simulink model "h2omnix_heading"  (R2022b)
settings: Solver=ode4  StartTime=0.0  StopTime=inf  FixedStep=0.05  RelTol=1e-3
values from neighbouring files (symbols this model uses):
  nu_max = [0.5,0.5,1]'    [parameters.m]
  nu_min = -nu_max    [parameters.m]
  pcKd = pcKd.*disable    [parameters.m]
  pcKp = pcKp.*disable    [parameters.m]
  vcKi = vcKi.*disable    [parameters.m]
  vcKp = vcKp.*disable    [parameters.m]
  vcKt = vcKt.*disable    [parameters.m]
  wn = 3*wpn/2    [parameters.m]
  wpn = [1.2, 1.2, 1]'    [parameters.m]
libraries: ros2lib x4, MarineRoboticsLib x3, MarineRoboticsLibEx x1, robotcorelib x1, matrix_library x1, simulink x1
settings Model: DataDictionary=ros2lib.sldd  Creator=dnad  LastModifiedBy=dnad

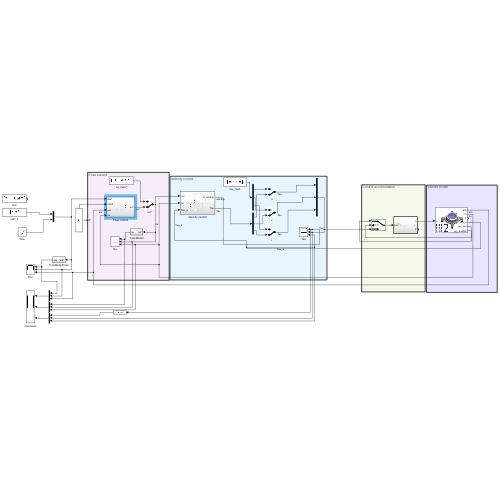
[thumbnail: Simulink's stored preview of the top-level diagram]
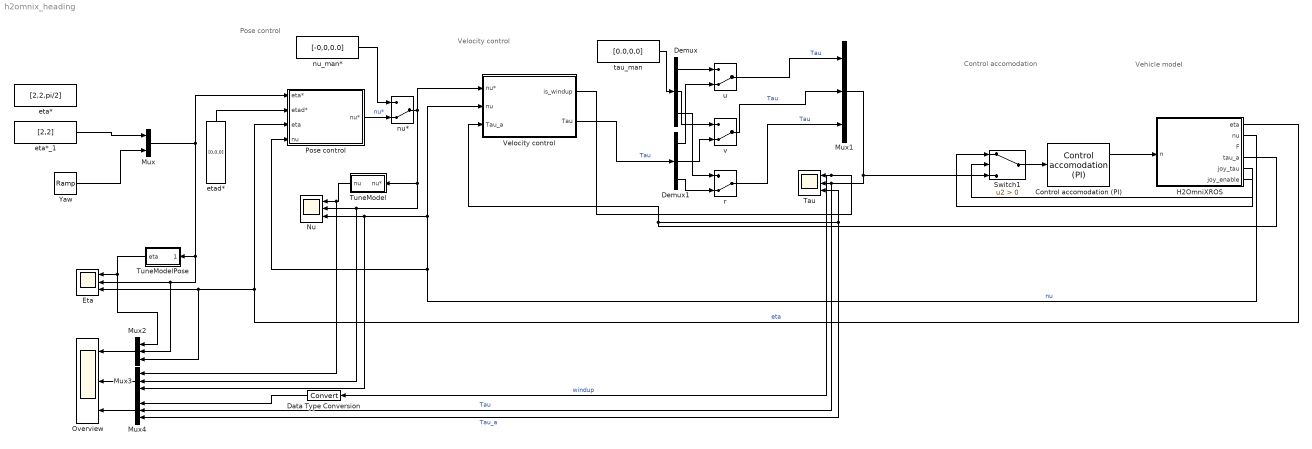
== system h2omnix_heading ==
  note: Control accomodation
  note: Vehicle model
  note: Pose control
  note: Velocity control
  Control accomodation (PI) : MarineRoboticsLibEx/Control accomodation (PI)  SystemSampleTime=-1  VariantActivationTime=update diagram  Latency=0  AutoFrameSizeCalculation=off
  Data Type Conversion : DataTypeConversion  SaturateOnIntegerOverflow=off  RndMeth=Floor
  Demux : Demux  Outputs=3
  Demux1 : Demux  Outputs=3
  Eta : Scope  NumInputPorts=3
  H2OmniXROS : Subsystem  AncestorBlock=MarineRoboticsLib/H2OmniXROS  mask{vehicle_name=krk, max_pwm=0.4, pwm_topic=/krk/pwm_out, joy_topic=/krk/joy, odometry_topic=/krk/odometry/filtered}
      mask prompts: vehicle_name "Vehicle name"; max_pwm "Maximum allowed PWM"; pwm_topic "Command"; joy_topic "Joystick"; odometry_topic "Odometry"
      mask init:
      | set_param(gcb, 'pwm_topic',strcat('/', vehicle_name, '/pwm_out'));
      |     set_param(gcb, 'odometry_topic', strcat('/', vehicle_name, '/odometry/filtered'));
      |     set_param(gcb, 'joy_topic', strcat('/', vehicle_name, '/joy'));
      settings: LibrarySourceBlock=MarineRoboticsLib/H2OmniXROS
      mask TypeOptions pwm_topic: PublishToROS/topic
      mask TypeOptions joy_topic: Subscribe2/topic
      mask TypeOptions odometry_topic: Subscribe1/topic
      mask DialogControl G1 Prompt: Topics
      mask Display: image('$imagefile'); % Use "Edit Image" on toolstrip to change.
  Mux : Mux  Inputs=2
  Mux{1..4} (4 alike) : Mux  Inputs=3
  Nu : Scope  NumInputPorts=3
  Overview : Scope  NumInputPorts=3
  Pose control : Subsystem
  Switch1 : Switch  Criteria=u2 > Threshold  SaturateOnIntegerOverflow=off  InputSameDT=off
  Tau : Scope  NumInputPorts=3
  TuneModel : Subsystem
  TuneModelPose : Subsystem
  Velocity control : Subsystem
  Yaw : simulink/Sources/Ramp  slope=0.5  start=0  InitialOutput=0
  eta* : Constant  Value=[2,2,pi/2]
  eta*_1 : Constant  Value=[2,2]
  etad* : Constant  Value=[0,0,0]
  nu* : ManualSwitch  CurrentSetting=0
  nu_man* : Constant  Value=[-0,0,0.0]
  r : ManualSwitch  CurrentSetting=0
  tau_man : Constant  Value=[0.0,0,0]
  u : ManualSwitch  CurrentSetting=0
  v : ManualSwitch  CurrentSetting=0
  wires:
  Switch1/1 -> Control accomodation (PI)/1
  Control accomodation (PI)/1 -> H2OmniXROS/1(n)
  H2OmniXROS/5(joy_tau) -> Switch1/1
  H2OmniXROS/6(joy_enable) -> Switch1/2
  TuneModelPose/1(eta) -> Mux2/1, Eta/1
  Velocity control/1(is_windup) -> Data Type Conversion/1, Tau/1  "windup"
  etad*/1 -> Pose control/2(etad*)
  Pose control/1(nu*) -> nu*/2  "nu*"
  eta*_1/1 -> Mux/1
  Mux1/1 -> Mux4/2, Tau/2, Switch1/3  "Tau"
  TuneModel/1(nu) -> Mux3/1, Nu/1
  nu_man*/1 -> nu*/1
  H2OmniXROS/1(eta) -> Pose control/3(eta), Mux2/3, Eta/3  "eta"
  H2OmniXROS/2(nu) -> Velocity control/2(nu), Mux3/3, Nu/3, Pose control/4(nu)  "nu"
  H2OmniXROS/4(tau_a) -> Velocity control/3(Tau_a), Mux4/3, Tau/3  "Tau_a"
  Yaw/1 -> Mux/2
  nu*/1 -> Mux3/2, Nu/2, TuneModel/1(nu*), Velocity control/1(nu*)
  Mux/1 -> Pose control/1(eta*), Mux2/2, Eta/2, TuneModelPose/1(eta*)
  tau_man/1 -> Demux/1
  Velocity control/2(Tau) -> Demux1/1  "Tau"
  Demux/1 -> u/1
  Demux1/1 -> u/2
  Demux/2 -> v/1
  Demux1/2 -> v/2
  Demux/3 -> r/1
  Demux1/3 -> r/2
  r/1 -> Mux1/3  "Tau"
  v/1 -> Mux1/2  "Tau"
  u/1 -> Mux1/1  "Tau"
  Mux2/1 -> Overview/1
  Mux3/1 -> Overview/2
  Mux4/1 -> Overview/3
  Data Type Conversion/1 -> Mux4/1

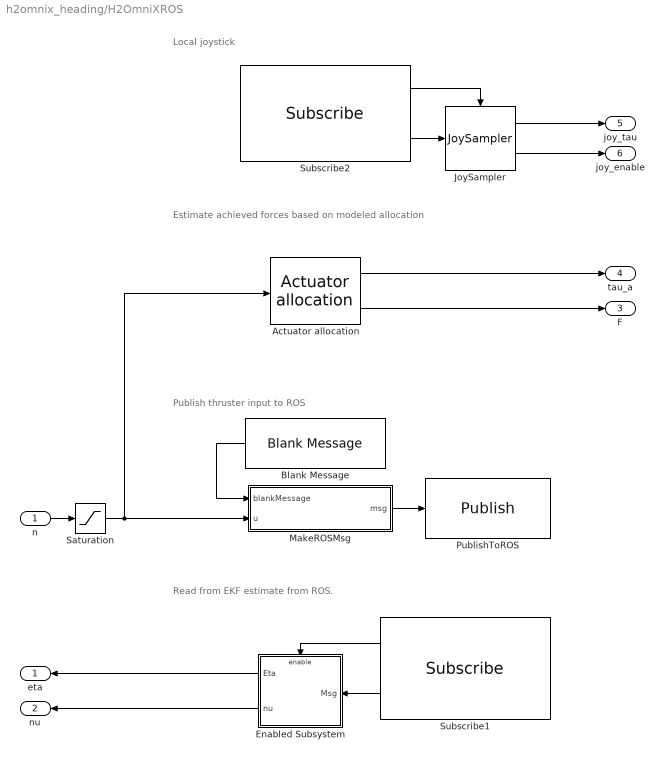
== system h2omnix_heading/H2OmniXROS ==
  note: Local joystick
  note: Read from EKF estimate from ROS.
  note: Publish thruster input to ROS
  note: Estimate achieved forces based on modeled allocation
  n : Inport
  Actuator allocation : MarineRoboticsLib/Actuator allocation  Tm=0  B="[0.25, 0.25, -0.25, -0.25; -0.25,  0.25, -0.25,  0.25; -0.25, 0.25, 0.25, -0.25]"  Keff=[1,1,1,1]
  Blank Message : ros2lib/Blank Message  messageClass=Message  entityType=std_msgs/Float32MultiArray  messageType=std_msgs/Float32MultiArray  SampleTime=0.05
  Enabled Subsystem : Subsystem  TreatAsAtomicUnit=on
  JoySampler : MarineRoboticsLib/JoyOverROS/JoySampler  SystemSampleTime=-1  VariantActivationTime=update diagram  Latency=0  AutoFrameSizeCalculation=off
  MakeROSMsg : MATLAB Function  TreatAsAtomicUnit=on  SystemSampleTime=0.05
  PublishToROS : ros2lib/Publish  topicSource=Select from ROS network  topic=/krk/pwm_out  messageType=std_msgs/Float32MultiArray  QOSHistory=Keep last  QOSDepth=1  QOSReliability=Reliable  QOSDurability=Volatile
  Saturation : Saturate  UpperLimit=max_pwm  LowerLimit=-max_pwm
  Subscribe1 : ros2lib/Subscribe  topicSource=Specify your own  topic=/krk/odometry/filtered  messageType=nav_msgs/Odometry  sampleTime=0.05  QOSHistory=Keep last  QOSDepth=1  QOSReliability=Reliable  QOSDurability=Volatile
  Subscribe2 : ros2lib/Subscribe  topicSource=Specify your own  topic=/krk/joy  messageType=sensor_msgs/Joy  sampleTime=0.05  QOSHistory=Keep last  QOSDepth=1  QOSReliability=Reliable  QOSDurability=Volatile
  eta : Outport
  nu : Outport  Port=2
  F : Outport  Port=3
  tau_a : Outport  Port=4
  joy_tau : Outport  Port=5
  joy_enable : Outport  Port=6
  wires:
  Saturation/1 -> Actuator allocation/1, MakeROSMsg/2(u)
  MakeROSMsg/1(msg) -> PublishToROS/1
  Subscribe1/2 -> Enabled Subsystem/1(Msg)
  Subscribe1/1 -> Enabled Subsystem/Enable
  Enabled Subsystem/1(Eta) -> eta/1
  Blank Message/1 -> MakeROSMsg/1(blankMessage)
  n/1 -> Saturation/1
  Enabled Subsystem/2(nu) -> nu/1
  Actuator allocation/2 -> F/1
  Actuator allocation/1 -> tau_a/1
  JoySampler/2 -> joy_enable/1
  Subscribe2/2 -> JoySampler/1
  JoySampler/1 -> joy_tau/1
  Subscribe2/1 -> JoySampler/Enable

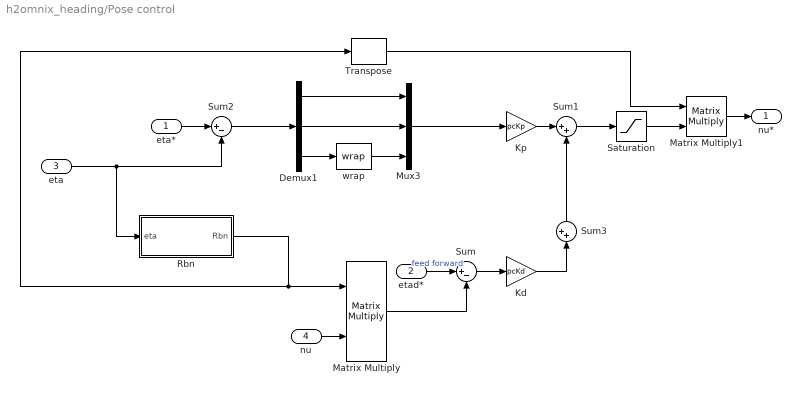
== system h2omnix_heading/Pose control ==
  eta* : Inport
  etad* : Inport  Port=2
  eta : Inport  Port=3
  nu : Inport  Port=4
  Demux1 : Demux  Outputs=3
  Kd : Gain  Gain=pcKd
  Kp : Gain  Gain=pcKp
  Matrix Multiply : Product  Multiplication=Matrix(*)
  Matrix Multiply1 : Product  Multiplication=Matrix(*)
  Mux3 : Mux  Inputs=3
  Rbn : MATLAB Function  TreatAsAtomicUnit=on
  Saturation : Saturate  UpperLimit=nu_max  LowerLimit=nu_min
  Sum : Sum  Inputs=|+-
  Sum1 : Sum  Inputs=|++
  Sum2 : Sum  Inputs=|+-
  Sum3 : Sum  Inputs=++|
  Transpose : matrix_library/Transpose
  wrap : MarineRoboticsLib/wrap  SystemSampleTime=-1  VariantActivationTime=update diagram  Latency=0  AutoFrameSizeCalculation=off
      settings: LibrarySourceBlock=|
      | simulink/User-Defined
      | Functions/MATLAB Function
  nu* : Outport
  wires:
  Sum/1 -> Kd/1
  eta/1 -> Rbn/1(eta), Sum2/2
  etad*/1 -> Sum/1  "feed forward"
  Kp/1 -> Sum1/1
  eta*/1 -> Sum2/1
  Sum2/1 -> Demux1/1
  Demux1/1 -> Mux3/1
  Demux1/2 -> Mux3/2
  Demux1/3 -> wrap/1
  wrap/1 -> Mux3/3
  Mux3/1 -> Kp/1
  Sum1/1 -> Saturation/1
  Sum3/1 -> Sum1/2
  Kd/1 -> Sum3/2
  Rbn/1(Rbn) -> Matrix Multiply/1, Transpose/1
  Matrix Multiply1/1 -> nu*/1
  nu/1 -> Matrix Multiply/2
  Matrix Multiply/1 -> Sum/2
  Saturation/1 -> Matrix Multiply1/2
  Transpose/1 -> Matrix Multiply1/1

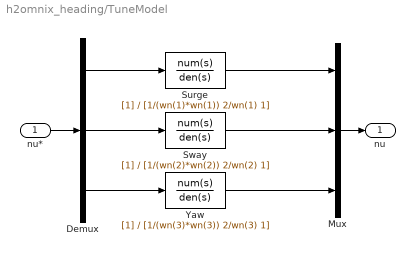
== system h2omnix_heading/TuneModel ==
  nu* : Inport
  Demux : Demux  Outputs=3
  Mux : Mux  Inputs=3
  Surge : TransferFcn  Denominator=[1/(wn(1)*wn(1)) 2/wn(1) 1]
  Sway : TransferFcn  Denominator=[1/(wn(2)*wn(2)) 2/wn(2) 1]
  Yaw : TransferFcn  Denominator=[1/(wn(3)*wn(3)) 2/wn(3) 1]
  nu : Outport
  wires:
  nu*/1 -> Demux/1
  Demux/1 -> Surge/1
  Surge/1 -> Mux/1
  Mux/1 -> nu/1
  Sway/1 -> Mux/2
  Demux/2 -> Sway/1
  Demux/3 -> Yaw/1
  Yaw/1 -> Mux/3

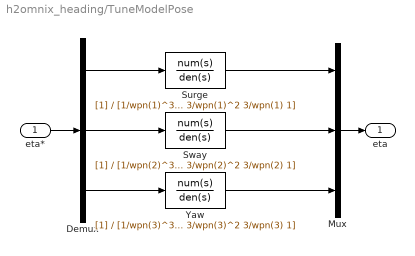
== system h2omnix_heading/TuneModelPose ==
  eta* : Inport
  Demux : Demux  Outputs=3
  Mux : Mux  Inputs=3
  Surge : TransferFcn  Denominator=[1/wpn(1)^3 3/wpn(1)^2 3/wpn(1) 1]
  Sway : TransferFcn  Denominator=[1/wpn(2)^3 3/wpn(2)^2 3/wpn(2) 1]
  Yaw : TransferFcn  Denominator=[1/wpn(3)^3 3/wpn(3)^2 3/wpn(3) 1]
  eta : Outport
  wires:
  eta*/1 -> Demux/1
  Demux/1 -> Surge/1
  Surge/1 -> Mux/1
  Mux/1 -> eta/1
  Sway/1 -> Mux/2
  Demux/2 -> Sway/1
  Demux/3 -> Yaw/1
  Yaw/1 -> Mux/3

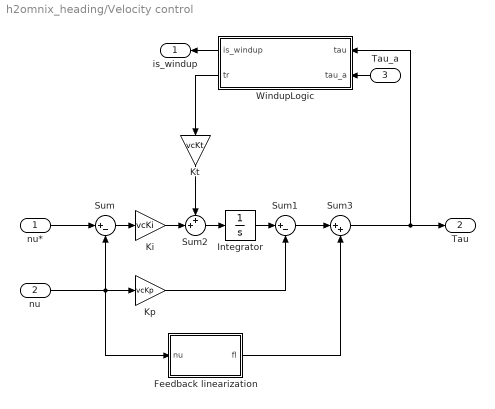
== system h2omnix_heading/Velocity control ==
  nu* : Inport
  nu : Inport  Port=2
  Tau_a : Inport  Port=3
  Feedback linearization : MATLAB Function  TreatAsAtomicUnit=on
  Integrator : Integrator
  Ki : Gain  Gain=vcKi
  Kp : Gain  Gain=vcKp
  Kt : Gain  Gain=vcKt
  Sum : Sum  Inputs=|+-
  Sum1 : Sum  Inputs=|+-
  Sum2 : Sum  Inputs=++|
  Sum3 : Sum  Inputs=|++
  WindupLogic : MATLAB Function  TreatAsAtomicUnit=on
  is_windup : Outport
  Tau : Outport  Port=2
  wires:
  Tau_a/1 -> WindupLogic/2(tau_a)
  nu/1 -> Feedback linearization/1(nu), Kp/1, Sum/2
  Integrator/1 -> Sum1/1
  nu*/1 -> Sum/1
  Sum/1 -> Ki/1
  Sum2/1 -> Integrator/1
  Kp/1 -> Sum1/2
  Ki/1 -> Sum2/2
  WindupLogic/1(is_windup) -> is_windup/1
  WindupLogic/2(tr) -> Kt/1
  Sum1/1 -> Sum3/1
  Sum3/1 -> WindupLogic/1(tau), Tau/1
  Feedback linearization/1(fl) -> Sum3/2
  Kt/1 -> Sum2/1

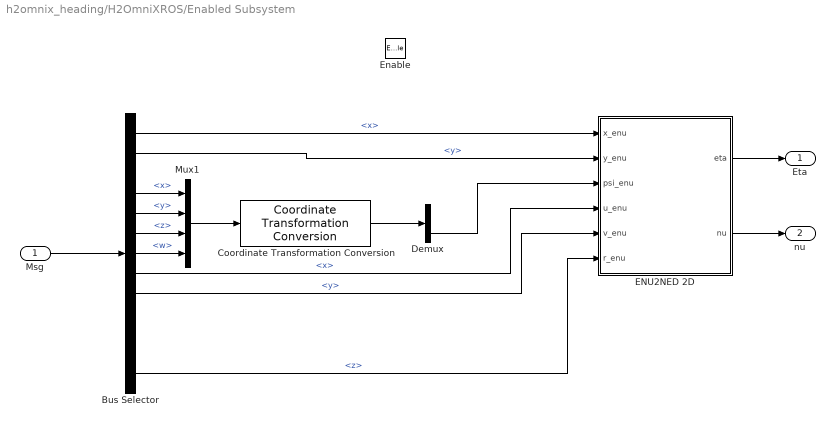
== system h2omnix_heading/H2OmniXROS/Enabled Subsystem ==
  Msg : Inport
  Enable : EnablePort
  Bus Selector : BusSelector  OutputSignals=pose.pose.position.x,pose.pose.position.y,pose.pose.position.z,pose.pose.orientation.x,pose.pose.orientation.y,pose.pose.orientation.z,pose.pose.orientation.w,twist.twist.linear.x,twist.twist.linear.y,twist.twist.linear.z,twist.twist.angular.x,twist.twist.angular.y,twist.twist.angular.z
  Coordinate Transformation Conversion : robotcorelib/Coordinate Transformation Conversion  InputRepresentation=Quaternion  InputEulerSequence=ZYX  ShowTrVecInputPort=on  OutputRepresentation=Euler Angles  OutputEulerSequence=ZYX  ShowTrVecOutputPort=on  SimulateUsing=Interpreted execution
      settings: LibrarySourceBlock=roslib/Utilities/Coordinate Transformation Conversion
  Demux : Demux  Outputs=3
  ENU2NED 2D : MATLAB Function  TreatAsAtomicUnit=on
  Mux1 : Mux
  Eta : Outport
  nu : Outport  Port=2
  wires:
  Msg/1 -> Bus Selector/1
  Bus Selector/4 -> Mux1/1  "<x>"
  Bus Selector/5 -> Mux1/2  "<y>"
  Bus Selector/6 -> Mux1/3  "<z>"
  Bus Selector/7 -> Mux1/4  "<w>"
  Mux1/1 -> Coordinate Transformation Conversion/1
  Bus Selector/2 -> ENU2NED 2D/2(y_enu)  "<y>"
  Bus Selector/1 -> ENU2NED 2D/1(x_enu)  "<x>"
  Coordinate Transformation Conversion/1 -> Demux/1
  Bus Selector/8 -> ENU2NED 2D/4(u_enu)  "<x>"
  Bus Selector/9 -> ENU2NED 2D/5(v_enu)  "<y>"
  Bus Selector/13 -> ENU2NED 2D/6(r_enu)  "<z>"
  ENU2NED 2D/1(eta) -> Eta/1
  ENU2NED 2D/2(nu) -> nu/1
  Demux/3 -> ENU2NED 2D/3(psi_enu)

== matlab function h2omnix_heading/Velocity control/Feedback linearization ==
  data: nu input; fl output
function fl = feedback_lin(nu)
Betaa = [0, 0, 0]';
fl = Betaa.*abs(nu).*nu;
end

== matlab function h2omnix_heading/Velocity control/WindupLogic ==
  data: tau input; is_windup output; tau_a input; tr output
function [is_windup, tr] = checkWindup(tau, tau_a)
% Consider the tracking within tolerances
tol = 0.01;
is_windup = abs(tau-tau_a)>tol & abs(tau)>0.1;
tr = is_windup.*(tau_a - tau);
end

== matlab function h2omnix_heading/Pose control/Rbn ==
  data: eta input; Rbn output
function Rbn = RotMatrix(eta)

cp = cos(eta(3));
sp = sin(eta(3));

Rbn = [cp -sp 0;
     sp  cp 0;
      0   0 1];

== matlab function h2omnix_heading/H2OmniXROS/Enabled Subsystem/ENU2NED 2D ==
  data: x_enu input; eta output; y_enu input; psi_enu input; u_enu input; v_enu input; r_enu input; nu output
function [eta, nu] = enu2ned2d(x_enu,y_enu,psi_enu,u_enu,v_enu,r_enu)
% Just do coordinate swap
psi_ned = pi/2-psi_enu;

psi_ned = mod(psi_ned, 2*pi);

if psi_ned > pi
   psi_ned = -2*pi + psi_ned;
elseif psi_ned <= -pi 
   psi_ned = 2*pi + psi_ned;
end


eta = [y_enu; x_enu; psi_ned];
nu = [u_enu; -v_enu; -r_enu;];

== matlab function h2omnix_heading/H2OmniXROS/MakeROSMsg ==
  data: blankMessage input; u input; msg output Bus: SL_Bus_std_msgs_Float32MultiArray
function msg  = assign_bus(blankMessage,u)

% blank message input
msg = blankMessage;

% assign pwm values into data field
msg.data(1:numel(u)) = reshape(u,[],1);

% all other fields must be assigned to complete the message
msg.data_SL_Info.CurrentLength = uint32(numel(u));
msg.layout.dim(1).size = uint32(size(u,1));
msg.layout.dim(2).size = uint32(size(u,2));
msg.layout.dim(1).stride = uint32(numel(u));
msg.layout.dim(2).stride = uint32(prod(size(u,2)));
